simulink model "FSM"  (R2025b)
settings: Solver=FixedStepAuto  StartTime=0.0  StopTime=inf  FixedStep=0.5  RelTol=1e-3
undefined symbols (not defined in the file): pose
libraries: ros2lib x12
settings Model: Creator=sarp  LastModifiedBy=sarp

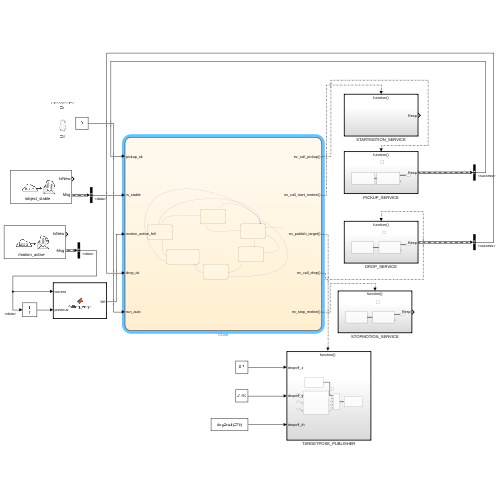
[thumbnail: Simulink's stored preview of the top-level diagram]
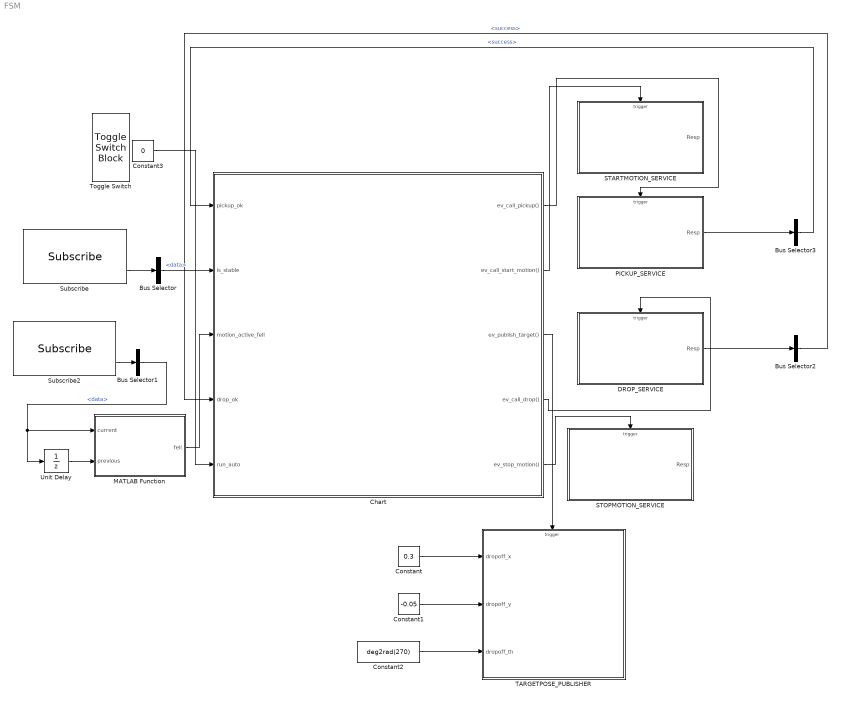
== system FSM ==
  Bus Selector : BusSelector  OutputSignals=data
  Bus Selector1 : BusSelector  OutputSignals=data
  Bus Selector2 : BusSelector  OutputSignals=success
  Bus Selector3 : BusSelector  OutputSignals=success
  Chart : Stateflow chart  TreatAsAtomicUnit=on
  Constant : Constant  Value=0.3
  Constant1 : Constant  Value=-0.05
  Constant2 : Constant  Value=deg2rad(270)
  Constant3 : Constant  Value=0
  DROP_SERVICE : Subsystem  TreatAsAtomicUnit=on
  MATLAB Function : MATLAB Function  TreatAsAtomicUnit=on
  PICKUP_SERVICE : Subsystem  TreatAsAtomicUnit=on
  STARTMOTION_SERVICE : Subsystem  TreatAsAtomicUnit=on
  STOPMOTION_SERVICE : Subsystem  TreatAsAtomicUnit=on
  Subscribe : ros2lib/Subscribe  topicSource=Select from ROS network  topic=/object_stable  messageType=std_msgs/Bool  sampleTime=-1  QOSHistory=Keep last  QOSDepth=10  QOSReliability=Reliable  QOSDurability=Volatile  QOSDeadline=Inf  QOSLifespan=Inf  QOSLiveliness=Automatic  QOSLeaseDuration=Inf  QOSAvoidROSNamespaceConventions=off
  Subscribe2 : ros2lib/Subscribe  topicSource=Select from ROS network  topic=/motion_active  messageType=std_msgs/Bool  sampleTime=-1  QOSHistory=Keep last  QOSDepth=10  QOSReliability=Reliable  QOSDurability=Volatile  QOSDeadline=Inf  QOSLifespan=Inf  QOSLiveliness=Automatic  QOSLeaseDuration=Inf  QOSAvoidROSNamespaceConventions=off
  TARGETPOSE_PUBLISHER : Subsystem  TreatAsAtomicUnit=on
  Toggle Switch : ToggleSwitchBlock
  Unit Delay : UnitDelay  SampleTime=-1  HasFrameUpgradeWarning=on
  wires:
  Chart/3(ev_publish_target()) -> TARGETPOSE_PUBLISHER/Trigger
  Chart/2(ev_call_start_motion()) -> STARTMOTION_SERVICE/Trigger
  Chart/1(ev_call_pickup()) -> PICKUP_SERVICE/Trigger
  Chart/4(ev_call_drop()) -> DROP_SERVICE/Trigger
  Subscribe/2 -> Bus Selector/1
  Bus Selector/1 -> Chart/2(is_stable)  "<data>"
  Subscribe2/2 -> Bus Selector1/1
  Bus Selector1/1 -> MATLAB Function/1(current), Unit Delay/1  "<data>"
  DROP_SERVICE/1(Resp) -> Bus Selector2/1
  Bus Selector2/1 -> Chart/4(drop_ok)  "<success>"
  Constant/1 -> TARGETPOSE_PUBLISHER/1(dropoff_x)
  Constant1/1 -> TARGETPOSE_PUBLISHER/2(dropoff_y)
  Constant2/1 -> TARGETPOSE_PUBLISHER/3(dropoff_th)
  Unit Delay/1 -> MATLAB Function/2(previous)
  MATLAB Function/1(fell) -> Chart/3(motion_active_fell)
  PICKUP_SERVICE/1(Resp) -> Bus Selector3/1
  Bus Selector3/1 -> Chart/1(pickup_ok)  "<success>"
  Constant3/1 -> Chart/5(run_auto)
  Chart/5(ev_stop_motion()) -> STOPMOTION_SERVICE/Trigger

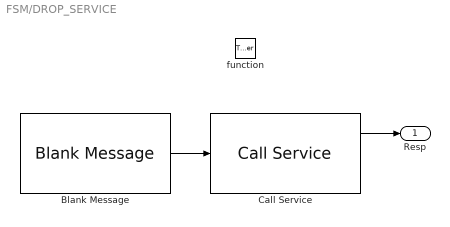
== system FSM/DROP_SERVICE ==
  function : TriggerPort  TriggerType=function-call  VariantControl=(inherit)
  Blank Message : ros2lib/Blank Message  messageClass=Service Request  entityType=std_srvs/Trigger  messageType=std_srvs/TriggerRequest  SampleTime=inf
  Call Service : ros2lib/Call Service  topicSource=Select from ROS network  service=/drop  serviceType=std_srvs/Trigger  connectionTimeout=5  ShowErrorCodeOutput=on  legacyBusStruct=off  QOSHistory=Keep last  QOSDepth=1  QOSReliability=Reliable  QOSDurability=Volatile  QOSDeadline=Inf  QOSLifespan=Inf  QOSLiveliness=Automatic  QOSLeaseDuration=Inf  QOSAvoidROSNamespaceConventions=off
  Resp : Outport
  wires:
  Call Service/1 -> Resp/1
  Blank Message/1 -> Call Service/1

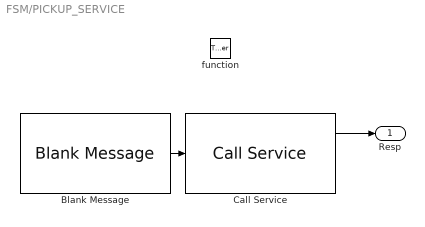
== system FSM/PICKUP_SERVICE ==
  function : TriggerPort  TriggerType=function-call  VariantControl=(inherit)
  Blank Message : ros2lib/Blank Message  messageClass=Service Request  entityType=std_srvs/Trigger  messageType=std_srvs/TriggerRequest  SampleTime=inf
  Call Service : ros2lib/Call Service  topicSource=Select from ROS network  service=/pickup  serviceType=std_srvs/Trigger  connectionTimeout=5  ShowErrorCodeOutput=on  legacyBusStruct=off  QOSHistory=Keep last  QOSDepth=1  QOSReliability=Reliable  QOSDurability=Volatile  QOSDeadline=Inf  QOSLifespan=Inf  QOSLiveliness=Automatic  QOSLeaseDuration=Inf  QOSAvoidROSNamespaceConventions=off
  Resp : Outport
  wires:
  Call Service/1 -> Resp/1
  Blank Message/1 -> Call Service/1

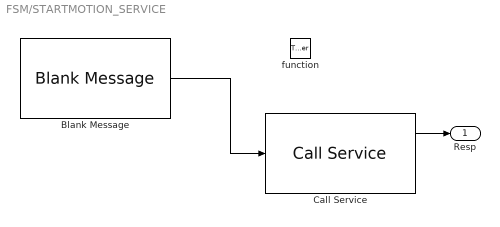
== system FSM/STARTMOTION_SERVICE ==
  function : TriggerPort  TriggerType=function-call  VariantControl=(inherit)
  Blank Message : ros2lib/Blank Message  messageClass=Service Request  entityType=std_srvs/Trigger  messageType=std_srvs/TriggerRequest  SampleTime=inf
  Call Service : ros2lib/Call Service  topicSource=Select from ROS network  service=/start_motion  serviceType=std_srvs/Trigger  connectionTimeout=5  ShowErrorCodeOutput=on  legacyBusStruct=off  QOSHistory=Keep last  QOSDepth=1  QOSReliability=Reliable  QOSDurability=Volatile  QOSDeadline=Inf  QOSLifespan=Inf  QOSLiveliness=Automatic  QOSLeaseDuration=Inf  QOSAvoidROSNamespaceConventions=off
  Resp : Outport
  wires:
  Call Service/1 -> Resp/1
  Blank Message/1 -> Call Service/1

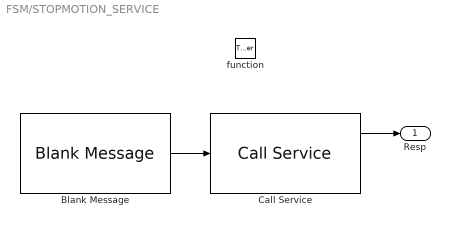
== system FSM/STOPMOTION_SERVICE ==
  function : TriggerPort  TriggerType=function-call  VariantControl=(inherit)
  Blank Message : ros2lib/Blank Message  messageClass=Service Request  entityType=std_srvs/Trigger  messageType=std_srvs/TriggerRequest  SampleTime=inf
  Call Service : ros2lib/Call Service  topicSource=Select from ROS network  service=/stop_motion  serviceType=std_srvs/Trigger  connectionTimeout=5  ShowErrorCodeOutput=on  legacyBusStruct=off  QOSHistory=Keep last  QOSDepth=1  QOSReliability=Reliable  QOSDurability=Volatile  QOSDeadline=Inf  QOSLifespan=Inf  QOSLiveliness=Automatic  QOSLeaseDuration=Inf  QOSAvoidROSNamespaceConventions=off
  Resp : Outport
  wires:
  Call Service/1 -> Resp/1
  Blank Message/1 -> Call Service/1

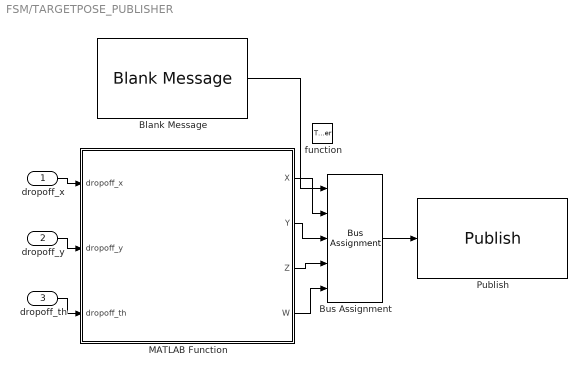
== system FSM/TARGETPOSE_PUBLISHER ==
  dropoff_x : Inport
  dropoff_y : Inport  Port=2
  dropoff_th : Inport  Port=3
  function : TriggerPort  TriggerType=function-call  VariantControl=(inherit)
  Blank Message : ros2lib/Blank Message  messageClass=Message  entityType=geometry_msgs/PoseStamped  messageType=geometry_msgs/PoseStamped  SampleTime=inf
  Bus Assignment : BusAssignment  AssignedSignals=pose.position.x,pose.position.y,pose.orientation.z,pose.orientation.w
  MATLAB Function : MATLAB Function  TreatAsAtomicUnit=on
  Publish : ros2lib/Publish  topicSource=Select from ROS network  topic=/target_pose  messageType=geometry_msgs/PoseStamped  QOSHistory=Keep last  QOSDepth=10  QOSReliability=Reliable  QOSDurability=Volatile  QOSDeadline=Inf  QOSLifespan=Inf  QOSLiveliness=Automatic  QOSLeaseDuration=Inf  QOSAvoidROSNamespaceConventions=off
  wires:
  dropoff_x/1 -> MATLAB Function/1(dropoff_x)
  dropoff_y/1 -> MATLAB Function/2(dropoff_y)
  dropoff_th/1 -> MATLAB Function/3(dropoff_th)
  Bus Assignment/1 -> Publish/1
  Blank Message/1 -> Bus Assignment/1
  MATLAB Function/1(X) -> Bus Assignment/2
  MATLAB Function/2(Y) -> Bus Assignment/3
  MATLAB Function/3(Z) -> Bus Assignment/4
  MATLAB Function/4(W) -> Bus Assignment/5

== matlab function FSM/MATLAB Function ==
  data: current input; fell output; previous input
function fell = falling_edge(current, previous)                          
  fell = (previous == true) && (current == false);                                 
end

== matlab function FSM/TARGETPOSE_PUBLISHER/MATLAB Function ==
  data: dropoff_x input; dropoff_y input; dropoff_th input; X output; Y output; Z output; W output
function [X,Y,Z,W ] = build_target_pose(dropoff_x, dropoff_y, dropoff_th)                            
    X         = double(dropoff_x);                                 
    Y         = double(dropoff_y);           
    Z      = double(sin(dropoff_th / 2));                       
    W      = double(cos(dropoff_th / 2)); 
end

== stateflow chart FSM/Chart ==
  state DROPOFF
    send(ev_call_drop);
  state IDLE
  state MOVTODROPOFF
    entry: send(ev_call_start_motion)
  state STABILIZING
  state PICKINGUP
    entry: send(ev_call_pickup);
  state MOVINGTOOBJECT
    entry: send(ev_call_start_motion)
  PICKINGUP -> IDLE [order 2] : [run_auto == 0]{send(ev_stop_motion)}
  MOVTODROPOFF -> IDLE [order 2] : [run_auto == 0]{send(ev_stop_motion)}
  DROPOFF -> IDLE [order 2] : [run_auto == 0]{send(ev_stop_motion)}
  MOVTODROPOFF -> DROPOFF [order 1] : [motion_active_fell==1]
  MOVINGTOOBJECT -> IDLE [order 2] : [run_auto == 0]{send(ev_stop_motion)}
  DROPOFF -> IDLE [order 1] : [drop_ok == 1]
  (default) -> IDLE
  STABILIZING -> IDLE [order 2] : [run_auto == 0]{send(ev_stop_motion)}
  IDLE -> STABILIZING : [run_auto ==1]
  PICKINGUP -> MOVTODROPOFF [order 1] : [pickup_ok==1]{send(ev_publish_target)}
  STABILIZING -> MOVINGTOOBJECT [order 1] : [is_stable ==1]
  MOVINGTOOBJECT -> PICKINGUP [order 1] : [motion_active_fell==1]
  data: pickup_ok input; is_stable input; motion_active_fell input; drop_ok input; run_auto input
  events: ev_call_pickup output FUNCTION_CALL_EVENT; ev_call_start_motion output FUNCTION_CALL_EVENT; ev_publish_target output FUNCTION_CALL_EVENT; ev_call_drop output FUNCTION_CALL_EVENT; ev_stop_motion output FUNCTION_CALL_EVENT
